simulink library "INT_PIntkVUs_VD"  (R2016b)
settings: Solver=VariableStepAuto  StartTime=0.0  StopTime=10.0  RelTol=1e-3
settings Model: Creator=Administrator  LastModifiedBy=Administrator

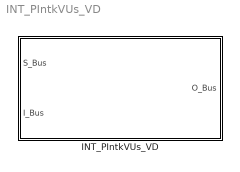
== system INT_PIntkVUs_VD ==
  INT_PIntkVUs_VD : Subsystem

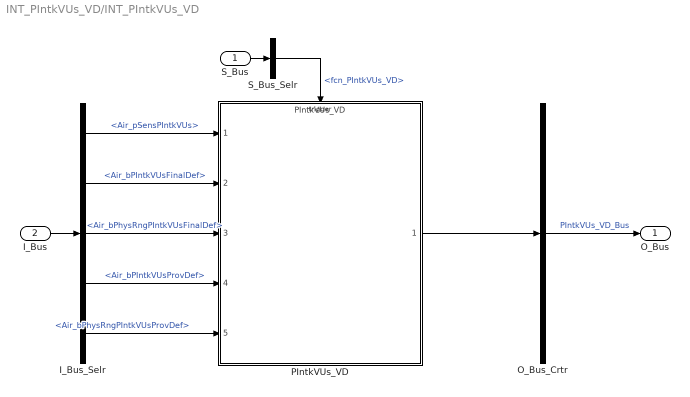
== system INT_PIntkVUs_VD/INT_PIntkVUs_VD ==
  S_Bus : Inport
  I_Bus : Inport  Port=2
  I_Bus_Selr : BusSelector  OutputSignals=Air_pSensPIntkVUs,Air_bPIntkVUsFinalDef,Air_bPhysRngPIntkVUsFinalDef,Air_bPIntkVUsProvDef,Air_bPhysRngPIntkVUsProvDef
  O_Bus_Crtr : BusCreator  Inputs=1
  PIntkVUs_VD : ModelReference  ModelNameDialog=PIntkVUs_VD  SimulationMode=Normal  ModelReferenceVersion=1.31  TriggerPortName=function  TriggerPortTriggerType=function-call  TriggerPortStatesWhenEnabling=held
  S_Bus_Selr : BusSelector  OutputSignals=fcn_PIntkVUs_VD
  O_Bus : Outport
  wires:
  S_Bus_Selr/1 -> PIntkVUs_VD/Trigger  "<fcn_PIntkVUs_VD>"
  S_Bus/1 -> S_Bus_Selr/1
  I_Bus/1 -> I_Bus_Selr/1
  I_Bus_Selr/1 -> PIntkVUs_VD/1  "<Air_pSensPIntkVUs>"
  I_Bus_Selr/2 -> PIntkVUs_VD/2  "<Air_bPIntkVUsFinalDef>"
  I_Bus_Selr/3 -> PIntkVUs_VD/3  "<Air_bPhysRngPIntkVUsFinalDef>"
  I_Bus_Selr/4 -> PIntkVUs_VD/4  "<Air_bPIntkVUsProvDef>"
  I_Bus_Selr/5 -> PIntkVUs_VD/5  "<Air_bPhysRngPIntkVUsProvDef>"
  O_Bus_Crtr/1 -> O_Bus/1  "PIntkVUs_VD_Bus"
  PIntkVUs_VD/1 -> O_Bus_Crtr/1
